simulink model "binary_inputs_model"  (Simulink 7.3)
settings: Solver=ode45  StartTime=0.0  StopTime=Tstop  RelTol=1e-3
values from neighbouring files (symbols this model uses):
  C = hybcon(S,Q,N,limits,refs)    [binary_inputs_sim.m]    (also in bm99benchmark.m; bm99norm2.m; bm99sim.m; exp2mld_mimo.m = lincon(model,'track',cost,interval,limits))
  Ts = 0.05    [bball.m]    (also in binary_inputs_sim.m = 1; bm99benchmark.m = 1; bm99norm2.m = 1; bm99sim.m = 1)
libraries: hyblib x2
settings Model: Creator=bemporad  LastModifiedBy=bemporad
settings DataIOCC: SignalLoggingName=sigsOut
settings DebuggingCC: SaveWithParameterizedLinksMsg=none  SignalResolutionControl=TryResolveAllWithWarning  SolverPrmCheckMsg=none  MultiTaskDSMMsg=warning  MultiTaskCondExecSysMsg=none  StrictBusMsg=None
settings HardwareCC: TargetUnknown=on
settings RTWCC: IncludeERTFirstTime=on

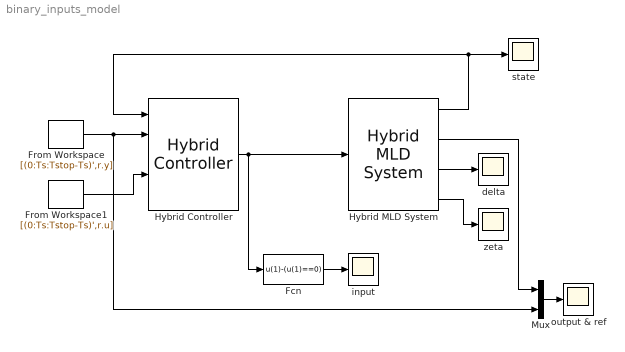
== system binary_inputs_model ==
  Fcn : Fcn  Expr=u(1)-(u(1)==0)
  From Workspace : FromWorkspace  VariableName=[(0:Ts:Tstop-Ts)',r.y]  SampleTime=Ts
  From Workspace1 : FromWorkspace  VariableName=[(0:Ts:Tstop-Ts)',r.u]  SampleTime=Ts
  Hybrid Controller : hyblib/Hybrid Controller  SystemSampleTime=-1  C=C  S=S  tilim=Inf
  Hybrid MLD System : hyblib/Hybrid MLD System  SystemSampleTime=-1  S=S  x0init=x0
  Mux : Mux  Inputs=2
  delta : Scope
  input : Scope
      settings: TimeRange=100  YMin=-1  YMax=1  SaveName=ScopeData2
  output & ref : Scope
      settings: TimeRange=100  SaveName=ScopeData4
  state : Scope
      settings: SaveName=ScopeData3
  zeta : Scope
  wires:
  Hybrid Controller/1 -> Hybrid MLD System/1, Fcn/1
  From Workspace/1 -> Hybrid Controller/2, Mux/2
  Mux/1 -> output & ref/1
  Hybrid MLD System/1 -> state/1, Hybrid Controller/1
  Hybrid MLD System/2 -> Mux/1
  Hybrid MLD System/3 -> delta/1
  Hybrid MLD System/4 -> zeta/1
  From Workspace1/1 -> Hybrid Controller/4
  Fcn/1 -> input/1
